simulink model "AWFG_Phase2_SIL"  (R2018a)
settings: Solver=ode3  StartTime=0.0  StopTime=0.1  RelTol=1e-3  EnableMultiTasking=on
libraries: simulink x7
Description:
  | AWFG_concept: This model explores the implementation concept
  | of an arbitrary waveform generator (AWFG) in a real-time target
  | platform with a combination of CPU and FPGA code.
  | This concepts aims at minimizing changes in the FPGA programming.
settings Model: Creator=Estra  LastModifiedBy=Talha Rao
settings DataIOCC: LimitDataPoints=on  SaveFormat=Array
settings OptimizationCC: DefaultParameterBehavior=Inlined  UseDivisionForNetSlopeComputation=on  UseFloatMulNetSlope=on  InlineInvariantSignals=on  PassReuseOutputArgsAs=Individual arguments  ExpressionDepthLimit=2147483647  ZeroExternalMemoryAtStartup=off  ZeroInternalMemoryAtStartup=off  NoFixptDivByZeroProtection=on  EfficientFloat2IntCast=on  LifeSpan=1
settings DebuggingCC: SignalInfNanChecking=warning  UnderspecifiedInitializationDetection=Classic  MergeDetectMultiDrivingBlocksExec=none  SolverPrmCheckMsg=warning  ParameterTunabilityLossMsg=error  UniqueDataStoreMsg=warning  AllowSymbolicDim=off  StateNameClashWarn=warning  SFUnexpectedBacktrackingDiag=warning  SFNoUnconditionalDefaultTransitionDiag=warning  SFExecutionAtInitializationDiag=none
settings HardwareCC: ProdLongLongMode=on
settings ModelReferenceCC: PropagateSignalLabelsOutOfModel=off
settings SFSimCC: MATLABDynamicMemAlloc=off
settings RTWCC: SystemTargetFile=ert.tlc  TemplateMakefile=ert_default_tmf  GenerateReport=on  IncludeHyperlinkInReport=on  LaunchReport=on  GenerateTraceInfo=on  GenerateTraceReport=on  GenerateTraceReportSl=on  GenerateTraceReportSf=on  GenerateTraceReportEml=on  GenerateCodeMetricsReport=on
settings CodeAppCC: ForceParamTrailComments=on  IgnoreCustomStorageClasses=off  OperatorAnnotations=on  SimulinkDataObjDesc=on  SFDataObjDesc=on  CustomSymbolStrGlobalVar=rt$N$M  CustomSymbolStrType=$N$M  CustomSymbolStrFcn=$N$M$F  CustomSymbolStrMacro=$N$M  InsertBlockDesc=on  StateflowObjectComments=on
settings ERTTargetCC: GenerateSampleERTMain=on  IncludeMdlTerminateFcn=off  CombineSignalStateStructs=on  SupportAbsoluteTime=off  SupportComplex=off  SupportNonInlinedSFcns=on  SupportVariableSizeSignals=on  InlinedParameterPlacement=NonHierarchical  ERTCustomFileTemplate=example_file_process.tlc  ERTFilePackagingFormat=CompactWithDataFile
settings ConfigComp: CovMetricSettings=dw  CovHtmlReporting=on  CovSaveCumulativeToWorkspaceVar=on  CovSaveSingleToWorkspaceVar=on  CovExternalEMLEnable=off

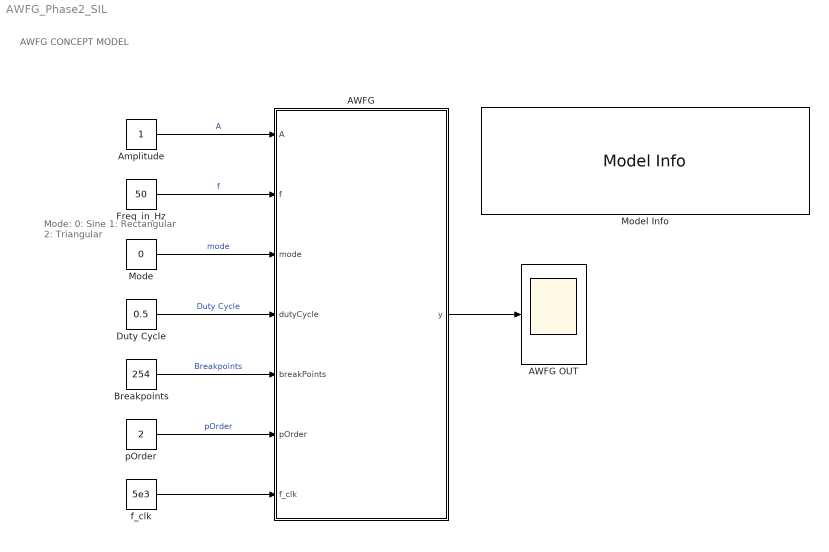
== system AWFG_Phase2_SIL ==
  note: AWFG CONCEPT MODEL
  note: Mode:
      | 0: Sine
      | 1: Rectangular
      | 2: Triangular
  AWFG : Subsystem
  AWFG OUT : Scope
  Amplitude : Constant  OutDataTypeStr=single
  Breakpoints : Constant  Value=254  OutDataTypeStr=single
  Duty Cycle : Constant  Value=0.5  OutDataTypeStr=single
  Freq_in_Hz : Constant  Value=50  OutDataTypeStr=single
  Mode : Constant  Value=0  OutDataTypeStr=single
  Model Info : simulink/Model-Wide Utilities/Model Info  Frame=on  DisplayStringWithTags=|  HorizontalTextAlignment=Left  LeftAlignmentValue=0.02
      | Model Info
      | Creator:       R. Estrada, FH JOANNEUM, 2018
      | Modified by: %<ModifiedBy>
      | Modify Date: %<ModifiedDate>
      | Version:%<ModelVersion>
      | Description:
      | %<Description>
  f_clk : Constant  Value=5e3
  pOrder : Constant  Value=2  OutDataTypeStr=single
  wires:
  AWFG/1(y) -> AWFG OUT/1
  Amplitude/1 -> AWFG/1(A)  "A"
  Freq_in_Hz/1 -> AWFG/2(f)  "f"
  Mode/1 -> AWFG/3(mode)  "mode"
  Duty Cycle/1 -> AWFG/4(dutyCycle)  "Duty Cycle"
  Breakpoints/1 -> AWFG/5(breakPoints)  "Breakpoints"
  pOrder/1 -> AWFG/6(pOrder)  "pOrder"
  f_clk/1 -> AWFG/7(f_clk)

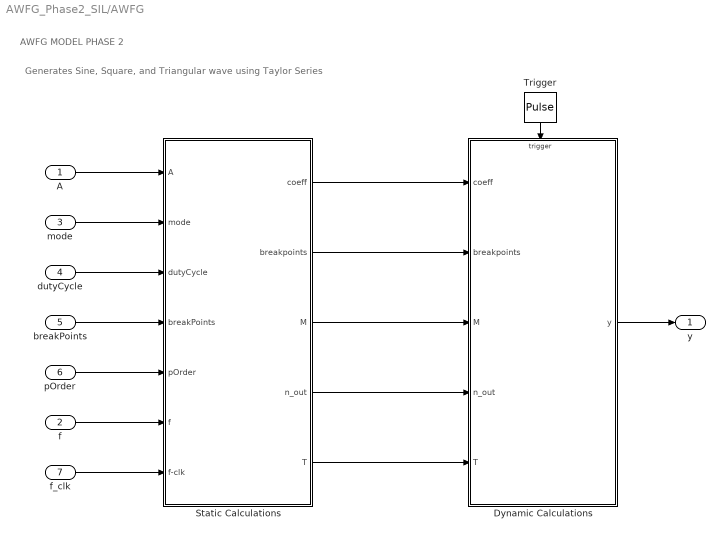
== system AWFG_Phase2_SIL/AWFG ==
  note: Generates Sine, Square, and Triangular wave using Taylor Series
  note: AWFG MODEL PHASE 2
  A : Inport
  f : Inport  Port=2
  mode : Inport  Port=3
  dutyCycle : Inport  Port=4
  breakPoints : Inport  Port=5
  pOrder : Inport  Port=6
  f_clk : Inport  Port=7
  Dynamic Calculations : Subsystem
  Static Calculations : Subsystem
  Trigger : DiscretePulseGenerator  PulseType=Time based  Period=1/5e3  PulseWidth=50
  y : Outport
  wires:
  Dynamic Calculations/1(y) -> y/1
  A/1 -> Static Calculations/1(A)
  mode/1 -> Static Calculations/2(mode)
  dutyCycle/1 -> Static Calculations/3(dutyCycle)
  breakPoints/1 -> Static Calculations/4(breakPoints)
  pOrder/1 -> Static Calculations/5(pOrder)
  f/1 -> Static Calculations/6(f)
  f_clk/1 -> Static Calculations/7(f-clk)
  Static Calculations/3(M) -> Dynamic Calculations/3(M)
  Static Calculations/4(n_out) -> Dynamic Calculations/4(n_out)
  Static Calculations/5(T) -> Dynamic Calculations/5(T)
  Static Calculations/1(coeff) -> Dynamic Calculations/1(coeff)
  Static Calculations/2(breakpoints) -> Dynamic Calculations/2(breakpoints)
  Trigger/1 -> Dynamic Calculations/Trigger

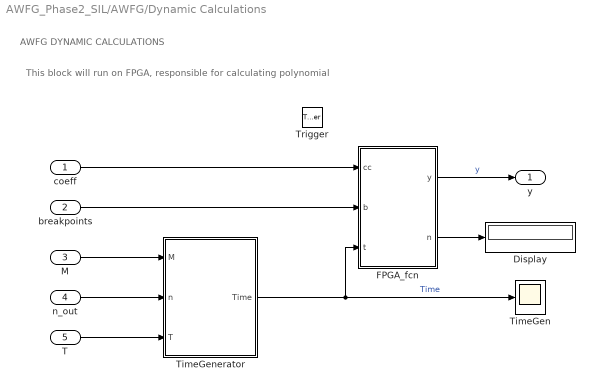
== system AWFG_Phase2_SIL/AWFG/Dynamic Calculations ==
  note: AWFG DYNAMIC CALCULATIONS
  note: This block will run on FPGA, responsible for calculating polynomial
  coeff : Inport
  breakpoints : Inport  Port=2
  M : Inport  Port=3
  n_out : Inport  Port=4
  T : Inport  Port=5
  Trigger : TriggerPort  VariantControl=Variant  PortDimensions=1
  Display : Display
  FPGA_fcn : MATLAB Function  TreatAsAtomicUnit=on
  TimeGen : Scope
  TimeGenerator : Subsystem
  y : Outport
  wires:
  FPGA_fcn/2(n) -> Display/1
  breakpoints/1 -> FPGA_fcn/2(b)
  FPGA_fcn/1(y) -> y/1  "y"
  TimeGenerator/1(Time) -> TimeGen/1, FPGA_fcn/3(t)  "Time"
  M/1 -> TimeGenerator/1(M)
  coeff/1 -> FPGA_fcn/1(cc)
  n_out/1 -> TimeGenerator/2(n)
  T/1 -> TimeGenerator/3(T)

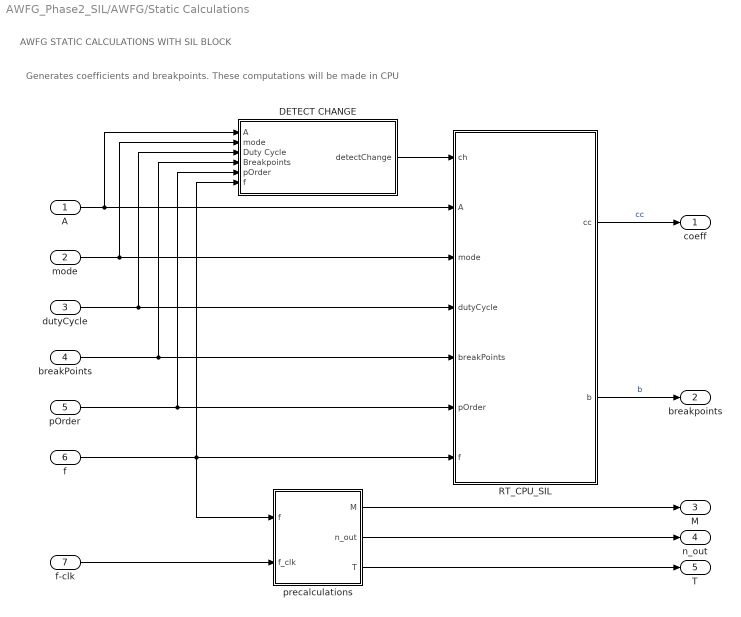
== system AWFG_Phase2_SIL/AWFG/Static Calculations ==
  note: AWFG STATIC CALCULATIONS WITH SIL BLOCK
  note: Generates coefficients and breakpoints. These computations will be made in CPU
  A : Inport
  mode : Inport  Port=2
  dutyCycle : Inport  Port=3
  breakPoints : Inport  Port=4
  pOrder : Inport  Port=5
  f : Inport  Port=6
  f-clk : Inport  Port=7
  DETECT CHANGE : Subsystem
  RT_CPU_SIL : Subsystem
      mask help: Simulink:masks:GenSFuncDesc_MD
      mask Help: eval('feval(''rtwprivate'',''rtwhelpview'',''rtw_sfcn_block'')');
  precalculations : Subsystem
  coeff : Outport
  breakpoints : Outport  Port=2
  M : Outport  Port=3
  n_out : Outport  Port=4
  T : Outport  Port=5
  wires:
  RT_CPU_SIL/2(b) -> breakpoints/1  "b"
  RT_CPU_SIL/1(cc) -> coeff/1  "cc"
  f/1 -> RT_CPU_SIL/7(f), precalculations/1(f), DETECT CHANGE/6(f)
  breakPoints/1 -> RT_CPU_SIL/5(breakPoints), DETECT CHANGE/4(Breakpoints)
  f-clk/1 -> precalculations/2(f_clk)
  A/1 -> RT_CPU_SIL/2(A), DETECT CHANGE/1(A)
  pOrder/1 -> RT_CPU_SIL/6(pOrder), DETECT CHANGE/5(pOrder)
  precalculations/2(n_out) -> n_out/1
  mode/1 -> RT_CPU_SIL/3(mode), DETECT CHANGE/2(mode)
  dutyCycle/1 -> RT_CPU_SIL/4(dutyCycle), DETECT CHANGE/3(Duty Cycle)
  DETECT CHANGE/1(detectChange) -> RT_CPU_SIL/1(ch)
  precalculations/3(T) -> T/1
  precalculations/1(M) -> M/1

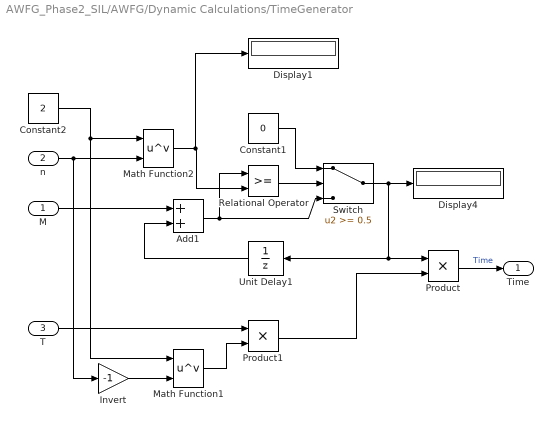
== system AWFG_Phase2_SIL/AWFG/Dynamic Calculations/TimeGenerator ==
  M : Inport
  n : Inport  Port=2
  T : Inport  Port=3
  Add1 : Sum
  Constant1 : Constant  Value=0
  Constant2 : Constant  Value=2
  Display1 : Display
  Display4 : Display
  Invert : Gain  Gain=-1
  Math Function1 : Math  Operator=pow  SaturateOnIntegerOverflow=on
  Math Function2 : Math  Operator=pow  SaturateOnIntegerOverflow=on
  Product : Product
  Product1 : Product
  Relational Operator : RelationalOperator  OutDataTypeStr=boolean  RndMeth=Nearest
  Switch : Switch  Threshold=0.5
  Unit Delay1 : UnitDelay  SampleTime=-1
  Time : Outport
  wires:
  T/1 -> Product1/1
  Invert/1 -> Math Function1/2
  Constant2/1 -> Math Function1/1, Math Function2/1
  n/1 -> Math Function2/2, Invert/1
  Math Function2/1 -> Relational Operator/2, Display1/1
  Math Function1/1 -> Product1/2
  Product/1 -> Time/1  "Time"
  Product1/1 -> Product/2
  Switch/1 -> Unit Delay1/1, Product/1, Display4/1
  Unit Delay1/1 -> Add1/2
  M/1 -> Add1/1
  Constant1/1 -> Switch/1
  Relational Operator/1 -> Switch/2
  Add1/1 -> Switch/3, Relational Operator/1

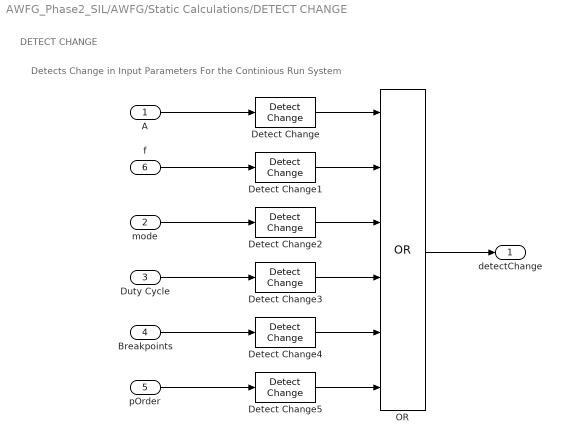
== system AWFG_Phase2_SIL/AWFG/Static Calculations/DETECT CHANGE ==
  note: Detects Change in Input Parameters For the Continious Run System
  note: DETECT CHANGE
  A : Inport
  mode : Inport  Port=2
  Duty Cycle : Inport  Port=3
  Breakpoints : Inport  Port=4
  pOrder : Inport  Port=5
  f : Inport  Port=6
  Detect Change{,1..5} (6 alike) : simulink/Logic and Bit Operations/Detect Change  vinit=0  OutDataTypeStr=boolean
  OR : Logic  Operator=OR  Inputs=6  AllPortsSameDT=off  OutDataTypeStr=boolean
  detectChange : Outport
  wires:
  Detect Change3/1 -> OR/4
  mode/1 -> Detect Change2/1
  Detect Change5/1 -> OR/6
  Detect Change1/1 -> OR/2
  Breakpoints/1 -> Detect Change4/1
  pOrder/1 -> Detect Change5/1
  Detect Change4/1 -> OR/5
  Detect Change2/1 -> OR/3
  Detect Change/1 -> OR/1
  Duty Cycle/1 -> Detect Change3/1
  f/1 -> Detect Change1/1
  A/1 -> Detect Change/1
  OR/1 -> detectChange/1

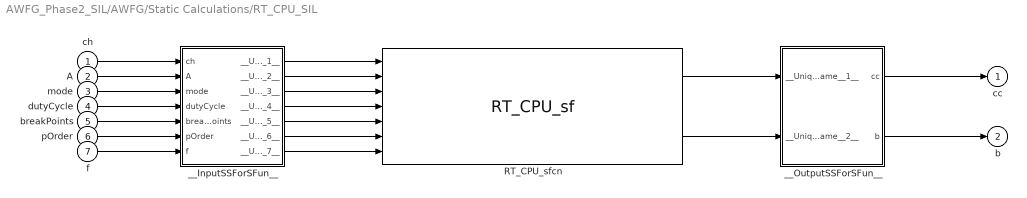
== system AWFG_Phase2_SIL/AWFG/Static Calculations/RT_CPU_SIL ==
  ch : Inport
  A : Inport  Port=2
  mode : Inport  Port=3
  dutyCycle : Inport  Port=4
  breakPoints : Inport  Port=5
  pOrder : Inport  Port=6
  f : Inport  Port=7
  RT_CPU_sfcn : S-Function  FunctionName=RT_CPU_sf  SFunctionModules=""  SFunctionDeploymentMode=off  EnableBusSupport=off  mask{rtw_sf_name=RT_CPU_sf, showVar=off}
      mask prompts: rtw_sf_name "Simulink:masks:GenSFuncName_MP"; showVar "Simulink:masks:GenSFuncShowModuleList_MP"
      mask help: Simulink:masks:GenSFuncDesc_MD
      mask init:
      | displist = '';
      | if ~strcmp(get_param(gcb, 'FunctionName'), rtw_sf_name);
      |   set_param(gcb, 'FunctionName', rtw_sf_name);
      | end
      | % Check if we are generating code
      | rtw_mode = false;
      | if strcmpi(get_param(bdroot(gcb),'SimulationStatus'),'Initializing')
      | 	rtw_mode = strcmpi(get_param(bdroot(gcb),'BuildingRTWCode'),'on') && ...
      | 		~strcmpi(get_param(bdroot(gcb),'TargetStyle'),'SimulationTarget');
      | end
      | if showVar || rtw_mode
      | 	if exist('rtwsfunc') == 2 | exist('rtwsfunc') == 6
      | 		tmplist = rtwsfunc(rtw_sf_name,gcb);
      | 		tmplist = DAStudio.message('Simulink:masks:GenSFuncListOfModules_IC', tmplist);
      | 	elseif showVar
      | 		tmplist1 = DAStudio.message('Simulink:masks:GenSFuncListOfModules_IC', '');
      |         tmplist2 = DAStudio.message('Simulink:masks:GenSFuncNotLicensed_IC');
      |         tmplist = [tmplist1 tmplist2];
      |  	end
      | end
      | if showVar
      |   displist = tmplist;
      | end
      settings: CopyFcn=|
      | if ~strcmp(get_param(gcb,'Linkstatus'),'none') && ...
      | ~strcmp(get_param(gcb,'Linkstatus'),'implicit')
      |   set_param(gcb,'LinkStatus','none');
      | end
      mask Help: eval('feval(''rtwprivate'',''rtwhelpview'',''rtw_sfcn_block'')');
      mask Display:
      | port_label('input',1,'ch');
      | port_label('input',2,'A');
      | port_label('input',3,'mode');
      | port_label('input',4,'dutyCycle');
      | port_label('input',5,'breakPoints');
      | port_label('input',6,'pOrder');
      | port_label('input',7,'f');
      | port_label('output',1,'cc');
      | port_label('output',2,'b');
  __InputSSForSFun__ : Subsystem
  __OutputSSForSFun__ : Subsystem
  cc : Outport
  b : Outport  Port=2
  wires:
  ch/1 -> __InputSSForSFun__/1(ch)
  A/1 -> __InputSSForSFun__/2(A)
  mode/1 -> __InputSSForSFun__/3(mode)
  dutyCycle/1 -> __InputSSForSFun__/4(dutyCycle)
  breakPoints/1 -> __InputSSForSFun__/5(breakPoints)
  pOrder/1 -> __InputSSForSFun__/6(pOrder)
  f/1 -> __InputSSForSFun__/7(f)
  __InputSSForSFun__/1(__UniqueOutportName__1__) -> RT_CPU_sfcn/1
  __InputSSForSFun__/2(__UniqueOutportName__2__) -> RT_CPU_sfcn/2
  __InputSSForSFun__/3(__UniqueOutportName__3__) -> RT_CPU_sfcn/3
  __InputSSForSFun__/4(__UniqueOutportName__4__) -> RT_CPU_sfcn/4
  __InputSSForSFun__/5(__UniqueOutportName__5__) -> RT_CPU_sfcn/5
  __InputSSForSFun__/6(__UniqueOutportName__6__) -> RT_CPU_sfcn/6
  __InputSSForSFun__/7(__UniqueOutportName__7__) -> RT_CPU_sfcn/7
  RT_CPU_sfcn/1 -> __OutputSSForSFun__/1(__UniqueInportName__1__)
  RT_CPU_sfcn/2 -> __OutputSSForSFun__/2(__UniqueInportName__2__)
  __OutputSSForSFun__/1(cc) -> cc/1
  __OutputSSForSFun__/2(b) -> b/1

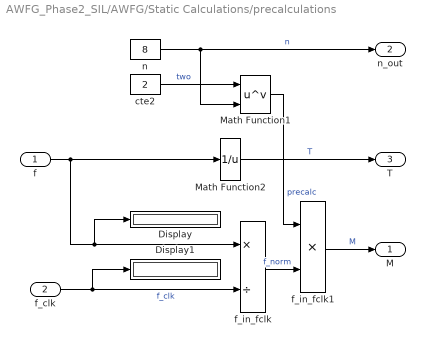
== system AWFG_Phase2_SIL/AWFG/Static Calculations/precalculations ==
  f : Inport
  f_clk : Inport  Port=2
  Display : Display
  Display1 : Display
  Math Function1 : Math  Operator=pow  SaturateOnIntegerOverflow=on
  Math Function2 : Math  Operator=reciprocal  SaturateOnIntegerOverflow=on
  cte2 : Constant  Value=2  SampleTime=-1
  f_in_fclk : Product  Inputs=*/
  f_in_fclk1 : Product  Inputs=**
  n : Constant  Value=8  SampleTime=-1
  M : Outport
  n_out : Outport  Port=2
  T : Outport  Port=3
  wires:
  cte2/1 -> Math Function1/1  "two"
  n/1 -> Math Function1/2, n_out/1  "n"
  Math Function1/1 -> f_in_fclk1/1  "precalc"
  Math Function2/1 -> T/1  "T"
  f_in_fclk1/1 -> M/1  "M"
  f_clk/1 -> f_in_fclk/2, Display1/1  "f_clk"
  f_in_fclk/1 -> f_in_fclk1/2  "f_norm"
  f/1 -> Math Function2/1, Display/1, f_in_fclk/1

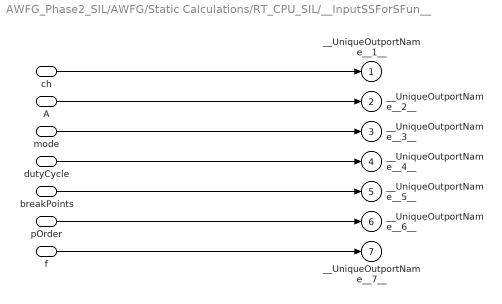
== system AWFG_Phase2_SIL/AWFG/Static Calculations/RT_CPU_SIL/__InputSSForSFun__ ==
  ch : Inport
  A : Inport  Port=2
  mode : Inport  Port=3
  dutyCycle : Inport  Port=4
  breakPoints : Inport  Port=5
  pOrder : Inport  Port=6
  f : Inport  Port=7
  __UniqueOutportName__1__ : Outport
  __UniqueOutportName__2__ : Outport  Port=2
  __UniqueOutportName__3__ : Outport  Port=3
  __UniqueOutportName__4__ : Outport  Port=4
  __UniqueOutportName__5__ : Outport  Port=5
  __UniqueOutportName__6__ : Outport  Port=6
  __UniqueOutportName__7__ : Outport  Port=7
  wires:
  ch/1 -> __UniqueOutportName__1__/1
  A/1 -> __UniqueOutportName__2__/1
  mode/1 -> __UniqueOutportName__3__/1
  dutyCycle/1 -> __UniqueOutportName__4__/1
  breakPoints/1 -> __UniqueOutportName__5__/1
  pOrder/1 -> __UniqueOutportName__6__/1
  f/1 -> __UniqueOutportName__7__/1

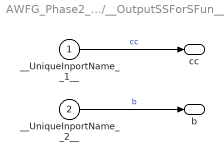
== system AWFG_Phase2_SIL/AWFG/Static Calculations/RT_CPU_SIL/__OutputSSForSFun__ ==
  __UniqueInportName__1__ : Inport
  __UniqueInportName__2__ : Inport  Port=2
  cc : Outport
  b : Outport  Port=2
  wires:
  __UniqueInportName__1__/1 -> cc/1  "cc"
  __UniqueInportName__2__/1 -> b/1  "b"

== matlab function AWFG_Phase2_SIL/AWFG/Dynamic Calculations/FPGA_fcn ==
  data: y output; cc input; b input; t input; n output
function [y,n]  = fcn(cc,b,t)
%% FPGA_simulation
%   This Embedded Matlab function solves a 4th-order polynomial output 
%       according to the coefficients and breaks points given as input. 
%
%
%       NOTE: In the final implementation this fcn will be placed at the    
%             FPGA
%       
%    Author: R. Estrada, FH JOANNEUM, 2018
%
%%

%#codegen

    n=size(cc,2)-1;
    i=find(b>t,1);       % find closest upper break point
    ii=max(i(1)-1,1);    % assign actual index for polynomial calculation

    % Calculate polynomial output according to actual relative time
    y=single(0);
    for j=0:1:n                
        y=y+cc(ii,j+1)*(t-b(ii))^j;
    end

end
